simulink model "SITL_gerador_codigo"  (R2015a)
settings: Solver=FixedStepDiscrete  StartTime=0.0  StopTime=tempofinal  FixedStep=Td  RelTol=1e-3
values from neighbouring files (symbols this model uses):
  cq = 2.4086*10^(-7)    (= 2.4086e-07)    [main_quad.m]
  ct = 1.4341*10^(-5)    (= 1.4341e-05)    [main_quad.m]
  d = 0.26    [main_quad.m]
  g = 9.8065    [main_quad.m]
  J = [Jxx,Jyy,Jzz,Jm]    [main_quad.m]
  k1 = 2.5    [main_quad.m]
  k2 = 6.2360    (= 6.236)    [main_quad.m]
  k3 = 6.2360    (= 6.236)    [main_quad.m]
  k4 = 0.4927    [main_quad.m]
  k5 = 1.6    [main_quad.m]
  k6 = 1.6    [main_quad.m]
  lambda1 = 1    [main_quad.m]
  lambda2 = 5    [main_quad.m]
  lambda3 = 5    [main_quad.m]
  lambda4 = 1/2    (= 0.5)    [main_quad.m]
  lambda5 = 1/4    (= 0.25)    [main_quad.m]
  lambda6 = 1/4    (= 0.25)    [main_quad.m]
  limit = [0.5 0.5 0.5 0.5]    [main_quad.m]
  limit_pos = [0.5 0.5]    [main_quad.m]
  m = 1.03    [main_quad.m]
  X = A(:,1)    [plot_resultados.m]
undefined symbols (not defined in the file or in its folder): selecting_parameters
libraries: dspnetwork x2, etargetslib x2
settings Model: ParamWorkspaceSource=ReferencedWorkspace  ExtModeTrigDuration=100  TunableVars=J,Td,cq,ct,d,g,k1,k2,k3,k4,k5,k6,lambda1,lambda2,lambda3,lambda4,lambda5,lambda6,limit,limit_pos,m  TunableVarsStorageClass=Auto,Auto,Auto,Auto,Auto,Auto,Auto,Auto,Auto,Auto,Auto,Auto,Auto,Auto,Auto,Auto,Auto,Auto,Auto,Auto,Auto  TunableVarsTypeQualifier=,,,,,,,,,,,,,,,,,,,,  Creator=Adriano  LastModifiedBy=Andre
settings OptimizationCC: InlineParams=on  EnhancedBackFolding=on  CachingGlobalReferences=on  StrengthReduction=on  OptimizeModelRefInitCode=on  LifeSpan=1  SimCompilerOptimization=on
settings DebuggingCC: UnderspecifiedInitializationDetection=Classic  MergeDetectMultiDrivingBlocksExec=none  SolverPrmCheckMsg=warning  StateNameClashWarn=warning
settings HardwareCC: ProdLargestAtomicInteger=Long  ProdLargestAtomicFloat=Double  ProdIntDivRoundTo=Zero  ProdEndianess=LittleEndian  ProdHWDeviceType=ARM Compatible->ARM Cortex
settings RTWCC: SystemTargetFile=ert.tlc  GenCodeOnly=on  GenerateMakefile=off  TemplateMakefile=ert_default_tmf  Description=Embedded Coder  GenerateReport=on  RTWVerbose=off  IncludeHyperlinkInReport=on  LaunchReport=on  RTWCompilerOptimization=on  CheckMdlBeforeBuild=Warning
settings CodeAppCC: IgnoreCustomStorageClasses=off
settings ERTTargetCC: ParMdlRefBuildCompliant=on  CompOptLevelCompliant=on  ConcurrentExecutionCompliant=on  ERTFirstTimeCompliant=on  SupportContinuousTime=off  SupportVariableSizeSignals=off  ModelStepFunctionPrototypeControlCompliant=on  CPPClassGenCompliant=on  InlinedParameterPlacement=Hierarchical  ERTCustomFileTemplate=example_file_process.tlc

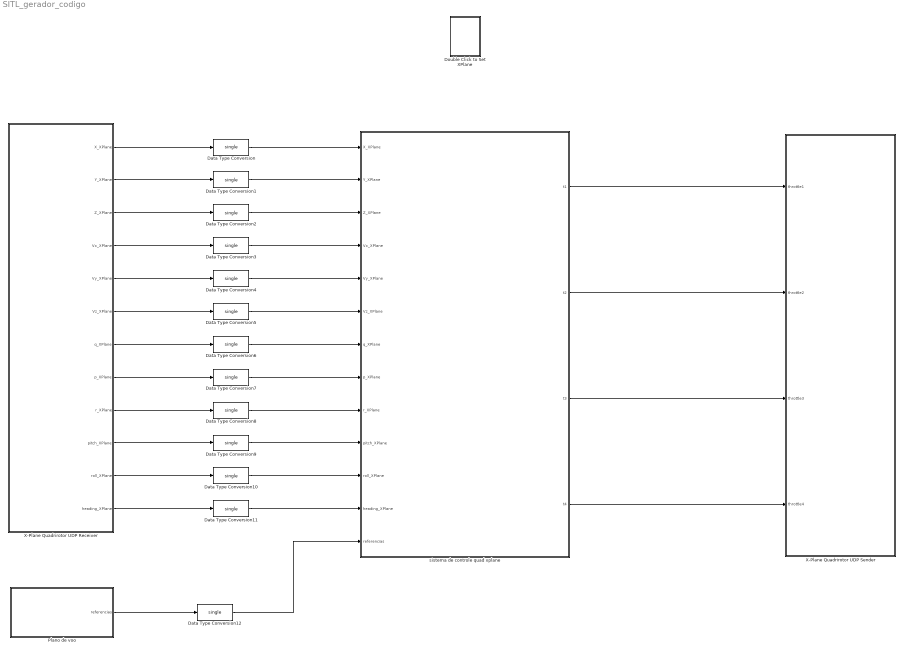
== system SITL_gerador_codigo ==
  Data Type Conversion{,1..12} (13 alike) : DataTypeConversion  OutDataTypeStr=single
  Double Click to Set XPlane : Subsystem  LoadFcn=selecting_parameters()
      settings: OpenFcn=selecting_parameters()
  Plano de voo : Subsystem
  X-Plane Quadrirotor UDP Receiver : Subsystem  AncestorBlock=X_Plane_Communication_Library/Fixed Wing/X-Plane Fixed Wing UDP Receiver  mask{ip_adress='127.0.0.1', port_number=49004}
      mask prompts: ip_adress "Local IP Adress (default: '127.0.0.1' )"; port_number "Output Port Number (defaut: '49004')"
      mask help: This block is configured to receiver data from a fixed wing aircraft on X-Plane Flight Simulator.
      mask Help: Contact adrianobittar@gmail.com
  X-Plane Quadrirotor UDP Sender : Subsystem  AncestorBlock=X_Plane_Communication_Library/Fixed Wing/X-Plane Fixed Wing UDP Sender  mask{ip_adress='127.0.0.1', port_number=49000}
      mask prompts: ip_adress "Local IP Adress (default: '127.0.0.1' )"; port_number "Output Port Number (defaut: '49000')"
      mask help: This block is configured to send data to a fixed wing aircraft on X-Plane Flight Simulator.
      mask Help: Contact adrianobittar@gmail.com
  sistema de controle quad xplane : Subsystem  DataTypeOverride=Single
  wires:
  X-Plane Quadrirotor UDP Receiver/1("X_XPlane ") -> Data Type Conversion/1
  X-Plane Quadrirotor UDP Receiver/2(Y_XPlane) -> Data Type Conversion1/1
  X-Plane Quadrirotor UDP Receiver/3(Z_XPlane) -> Data Type Conversion2/1
  X-Plane Quadrirotor UDP Receiver/4(Vx_XPlane) -> Data Type Conversion3/1
  X-Plane Quadrirotor UDP Receiver/5(Vy_XPlane) -> Data Type Conversion4/1
  X-Plane Quadrirotor UDP Receiver/6(Vz_XPlane) -> Data Type Conversion5/1
  X-Plane Quadrirotor UDP Receiver/7(q_XPlane) -> Data Type Conversion6/1
  X-Plane Quadrirotor UDP Receiver/8(p_XPlane) -> Data Type Conversion7/1
  X-Plane Quadrirotor UDP Receiver/9(r_XPlane) -> Data Type Conversion8/1
  X-Plane Quadrirotor UDP Receiver/10(pitch_XPlane) -> Data Type Conversion9/1
  X-Plane Quadrirotor UDP Receiver/11(roll_XPlane) -> Data Type Conversion10/1
  X-Plane Quadrirotor UDP Receiver/12(heading_XPlane) -> Data Type Conversion11/1
  Plano de voo/1("referencias ") -> Data Type Conversion12/1
  sistema de controle quad xplane/1(t1) -> X-Plane Quadrirotor UDP Sender/1(throttle1)
  sistema de controle quad xplane/2(t2) -> X-Plane Quadrirotor UDP Sender/2(throttle2)
  sistema de controle quad xplane/3(t3) -> X-Plane Quadrirotor UDP Sender/3(throttle3)
  sistema de controle quad xplane/4(t4) -> X-Plane Quadrirotor UDP Sender/4(throttle4)
  Data Type Conversion/1 -> sistema de controle quad xplane/1(X_XPlane)
  Data Type Conversion1/1 -> sistema de controle quad xplane/2(Y_XPlane)
  Data Type Conversion2/1 -> sistema de controle quad xplane/3(Z_XPlane)
  Data Type Conversion3/1 -> sistema de controle quad xplane/4(Vx_XPlane)
  Data Type Conversion4/1 -> sistema de controle quad xplane/5(Vy_XPlane)
  Data Type Conversion6/1 -> sistema de controle quad xplane/7(q_XPlane)
  Data Type Conversion5/1 -> sistema de controle quad xplane/6(Vz_XPlane)
  Data Type Conversion7/1 -> sistema de controle quad xplane/8(p_XPlane)
  Data Type Conversion9/1 -> sistema de controle quad xplane/10(pitch_XPlane)
  Data Type Conversion8/1 -> sistema de controle quad xplane/9(r_XPlane)
  Data Type Conversion10/1 -> sistema de controle quad xplane/11(roll_XPlane)
  Data Type Conversion11/1 -> sistema de controle quad xplane/12(heading_XPlane)
  Data Type Conversion12/1 -> sistema de controle quad xplane/13(referencias)

== system SITL_gerador_codigo/Double Click to Set XPlane ==

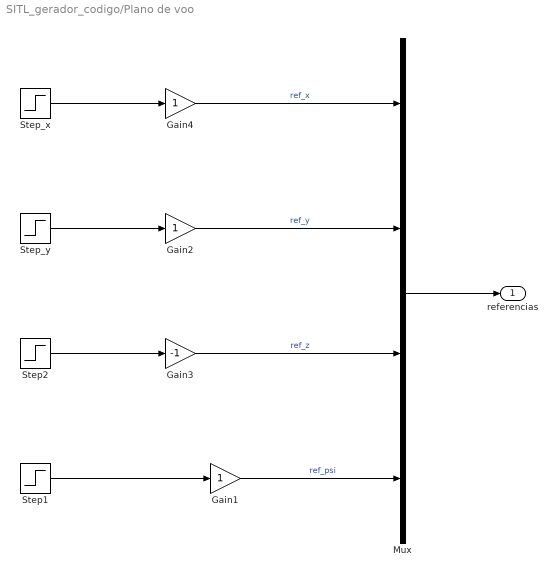
== system SITL_gerador_codigo/Plano de voo ==
  Gain1 : Gain
  Gain2 : Gain
  Gain3 : Gain  Gain=-1
  Gain4 : Gain
  Mux : Mux
  Step1 : Step  Time=30  After=150*pi/180  SampleTime=0
  Step2 : Step  Time=0  After=6  SampleTime=0
  Step_x : Step  Time=20  After=15  SampleTime=0
  Step_y : Step  Time=10  After=15  SampleTime=0
  "referencias " : Outport
  wires:
  Mux/1 -> "referencias "/1
  Gain3/1 -> Mux/3  "ref_z"
  Gain2/1 -> Mux/2  "ref_y"
  Gain4/1 -> Mux/1  "ref_x"
  Gain1/1 -> Mux/4  "ref_psi"
  Step1/1 -> Gain1/1
  Step2/1 -> Gain3/1
  Step_y/1 -> Gain2/1
  Step_x/1 -> Gain4/1

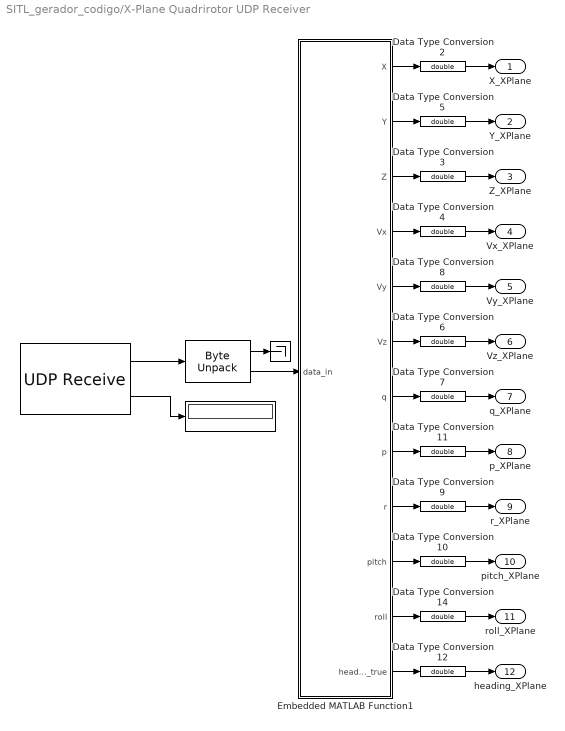
== system SITL_gerador_codigo/X-Plane Quadrirotor UDP Receiver ==
  " " : Display
  " " : Terminator
  "    " : dspnetwork/UDP Receive  localURL='0.0.0.0'  localPort=port_number  remoteURL=ip_adress  remotePort=-1  recvBufferSize=8192  dims=113  signalDatatype=uint8  isVarSize=off  showBlockingTime=on  blockingTime=1  sampletime=0.02  blockPlatform=WINDOWS
  "     " : etargetslib/Byte Unpack  dimensions={5,[9,3]}  datatypes={'uint8','single'}  byteAlign=1
  Data Type Conversion{2..12,14} (12 alike) : DataTypeConversion  OutDataTypeStr=double  SaturateOnIntegerOverflow=on
  Embedded MATLAB Function1 : MATLAB Function  TreatAsAtomicUnit=on
  "X_XPlane " : Outport
  Y_XPlane : Outport  Port=2
  Z_XPlane : Outport  Port=3
  Vx_XPlane : Outport  Port=4
  Vy_XPlane : Outport  Port=5
  Vz_XPlane : Outport  Port=6
  q_XPlane : Outport  Port=7
  p_XPlane : Outport  Port=8
  r_XPlane : Outport  Port=9
  pitch_XPlane : Outport  Port=10
  roll_XPlane : Outport  Port=11
  heading_XPlane : Outport  Port=12
  wires:
  Data Type Conversion11/1 -> p_XPlane/1
  Data Type Conversion14/1 -> roll_XPlane/1
  Data Type Conversion12/1 -> heading_XPlane/1
  Data Type Conversion7/1 -> q_XPlane/1
  Data Type Conversion6/1 -> Vz_XPlane/1
  Data Type Conversion4/1 -> Vx_XPlane/1
  Data Type Conversion3/1 -> Z_XPlane/1
  Data Type Conversion8/1 -> Vy_XPlane/1
  Data Type Conversion5/1 -> Y_XPlane/1
  Data Type Conversion2/1 -> "X_XPlane "/1
  Embedded MATLAB Function1/1(X) -> Data Type Conversion2/1
  Embedded MATLAB Function1/2(Y) -> Data Type Conversion5/1
  Embedded MATLAB Function1/3(Z) -> Data Type Conversion3/1
  Embedded MATLAB Function1/4(Vx) -> Data Type Conversion4/1
  Embedded MATLAB Function1/5(Vy) -> Data Type Conversion8/1
  Embedded MATLAB Function1/6(Vz) -> Data Type Conversion6/1
  Embedded MATLAB Function1/7(q) -> Data Type Conversion7/1
  Embedded MATLAB Function1/8(p) -> Data Type Conversion11/1
  Embedded MATLAB Function1/9(r) -> Data Type Conversion9/1
  Embedded MATLAB Function1/10(pitch) -> Data Type Conversion10/1
  Embedded MATLAB Function1/11(roll) -> Data Type Conversion14/1
  Embedded MATLAB Function1/12(heading_true) -> Data Type Conversion12/1
  "     "/1 -> " "/1
  "    "/2 -> " "/1
  Data Type Conversion10/1 -> pitch_XPlane/1
  "    "/1 -> "     "/1
  Data Type Conversion9/1 -> r_XPlane/1
  "     "/2 -> Embedded MATLAB Function1/1(data_in)

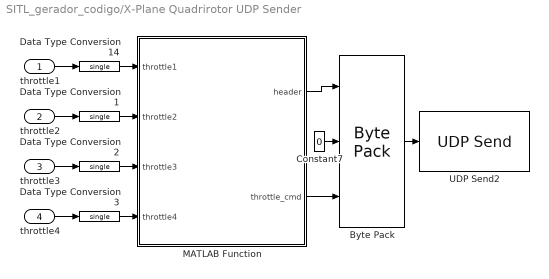
== system SITL_gerador_codigo/X-Plane Quadrirotor UDP Sender ==
  throttle1 : Inport
  throttle2 : Inport  Port=2
  throttle3 : Inport  Port=3
  throttle4 : Inport  Port=4
  Byte Pack : etargetslib/Byte Pack  datatypes={'single','uint8','single'}  byteAlign=1
  Constant7 : Constant  Value=0  OutDataTypeStr=uint8
  Data Type Conversion{1..3,14} (4 alike) : DataTypeConversion  OutDataTypeStr=single  SaturateOnIntegerOverflow=on
  MATLAB Function : MATLAB Function  TreatAsAtomicUnit=on
  UDP Send2 : dspnetwork/UDP Send  remoteURL=ip_adress  remotePort=port_number  localURL='255.255.255.255'  localPortSource=Automatically determine  localPort=-1  sampletime=-1  blockPlatform=HOST  separateLengthPort=0
  wires:
  Byte Pack/1 -> UDP Send2/1
  MATLAB Function/1(header) -> Byte Pack/1
  Data Type Conversion14/1 -> MATLAB Function/1(throttle1)
  throttle1/1 -> Data Type Conversion14/1
  Constant7/1 -> Byte Pack/2
  Data Type Conversion1/1 -> MATLAB Function/2(throttle2)
  Data Type Conversion2/1 -> MATLAB Function/3(throttle3)
  Data Type Conversion3/1 -> MATLAB Function/4(throttle4)
  throttle2/1 -> Data Type Conversion1/1
  throttle3/1 -> Data Type Conversion2/1
  throttle4/1 -> Data Type Conversion3/1
  MATLAB Function/2(throttle_cmd) -> Byte Pack/3

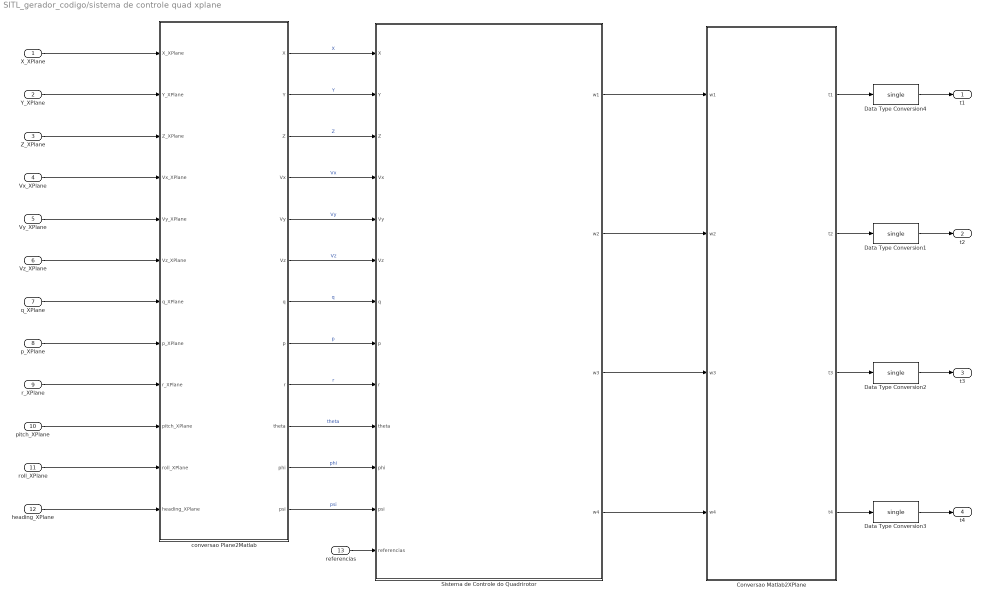
== system SITL_gerador_codigo/sistema de controle quad xplane ==
  X_XPlane : Inport
  Y_XPlane : Inport  Port=2
  Z_XPlane : Inport  Port=3
  Vx_XPlane : Inport  Port=4
  Vy_XPlane : Inport  Port=5
  Vz_XPlane : Inport  Port=6
  q_XPlane : Inport  Port=7
  p_XPlane : Inport  Port=8
  r_XPlane : Inport  Port=9
  pitch_XPlane : Inport  Port=10
  roll_XPlane : Inport  Port=11
  heading_XPlane : Inport  Port=12
  referencias : Inport  Port=13
  Conversao Matlab2XPlane : Subsystem
  Data Type Conversion{1..4} (4 alike) : DataTypeConversion  OutDataTypeStr=single
  Sistema de Controle do Quadrirotor : Subsystem
  conversao Plane2Matlab : Subsystem
  t1 : Outport
  t2 : Outport  Port=2
  t3 : Outport  Port=3
  t4 : Outport  Port=4
  wires:
  pitch_XPlane/1 -> conversao Plane2Matlab/10(pitch_XPlane)
  X_XPlane/1 -> conversao Plane2Matlab/1(X_XPlane)
  Y_XPlane/1 -> conversao Plane2Matlab/2(Y_XPlane)
  Z_XPlane/1 -> conversao Plane2Matlab/3(Z_XPlane)
  Vx_XPlane/1 -> conversao Plane2Matlab/4(Vx_XPlane)
  Vy_XPlane/1 -> conversao Plane2Matlab/5(Vy_XPlane)
  p_XPlane/1 -> conversao Plane2Matlab/8(p_XPlane)
  roll_XPlane/1 -> conversao Plane2Matlab/11(roll_XPlane)
  r_XPlane/1 -> conversao Plane2Matlab/9(r_XPlane)
  Vz_XPlane/1 -> conversao Plane2Matlab/6(Vz_XPlane)
  heading_XPlane/1 -> conversao Plane2Matlab/12(heading_XPlane)
  q_XPlane/1 -> conversao Plane2Matlab/7(q_XPlane)
  Sistema de Controle do Quadrirotor/3(w3) -> Conversao Matlab2XPlane/3(w3)
  Sistema de Controle do Quadrirotor/4(w4) -> Conversao Matlab2XPlane/4(w4)
  Sistema de Controle do Quadrirotor/2(w2) -> Conversao Matlab2XPlane/2(w2)
  Sistema de Controle do Quadrirotor/1(w1) -> Conversao Matlab2XPlane/1(w1)
  conversao Plane2Matlab/12(psi) -> Sistema de Controle do Quadrirotor/12(psi)  "psi"
  conversao Plane2Matlab/11(phi) -> Sistema de Controle do Quadrirotor/11(phi)  "phi"
  conversao Plane2Matlab/10(theta) -> Sistema de Controle do Quadrirotor/10(theta)  "theta"
  conversao Plane2Matlab/9(r) -> Sistema de Controle do Quadrirotor/9(r)  "r"
  conversao Plane2Matlab/8(p) -> Sistema de Controle do Quadrirotor/8(p)  "p"
  conversao Plane2Matlab/7(q) -> Sistema de Controle do Quadrirotor/7(q)  "q"
  conversao Plane2Matlab/6(Vz) -> Sistema de Controle do Quadrirotor/6(Vz)  "Vz"
  conversao Plane2Matlab/5(Vy) -> Sistema de Controle do Quadrirotor/5(Vy)  "Vy"
  conversao Plane2Matlab/4(Vx) -> Sistema de Controle do Quadrirotor/4(Vx)  "Vx"
  conversao Plane2Matlab/3(Z) -> Sistema de Controle do Quadrirotor/3(Z)  "Z"
  conversao Plane2Matlab/2(Y) -> Sistema de Controle do Quadrirotor/2(Y)  "Y"
  conversao Plane2Matlab/1("X ") -> Sistema de Controle do Quadrirotor/1(X)  "X"
  Conversao Matlab2XPlane/1(t1) -> Data Type Conversion4/1
  Conversao Matlab2XPlane/2(t2) -> Data Type Conversion1/1
  Conversao Matlab2XPlane/3(t3) -> Data Type Conversion2/1
  Conversao Matlab2XPlane/4(t4) -> Data Type Conversion3/1
  referencias/1 -> Sistema de Controle do Quadrirotor/13(referencias)
  Data Type Conversion4/1 -> t1/1
  Data Type Conversion1/1 -> t2/1
  Data Type Conversion2/1 -> t3/1
  Data Type Conversion3/1 -> t4/1

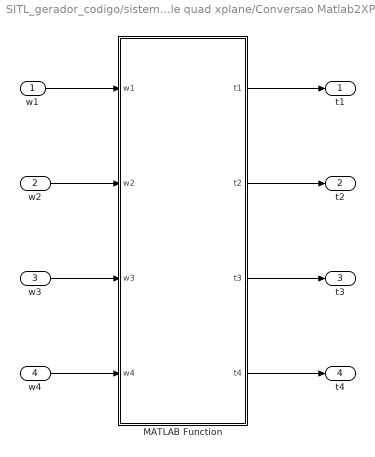
== system SITL_gerador_codigo/sistema de controle quad xplane/Conversao Matlab2XPlane ==
  w1 : Inport
  w2 : Inport  Port=2
  w3 : Inport  Port=3
  w4 : Inport  Port=4
  MATLAB Function : MATLAB Function  TreatAsAtomicUnit=on
  t1 : Outport
  t2 : Outport  Port=2
  t3 : Outport  Port=3
  t4 : Outport  Port=4
  wires:
  w1/1 -> MATLAB Function/1(w1)
  w2/1 -> MATLAB Function/2(w2)
  w3/1 -> MATLAB Function/3(w3)
  w4/1 -> MATLAB Function/4(w4)
  MATLAB Function/1(t1) -> t1/1
  MATLAB Function/2(t2) -> t2/1
  MATLAB Function/3(t3) -> t3/1
  MATLAB Function/4(t4) -> t4/1

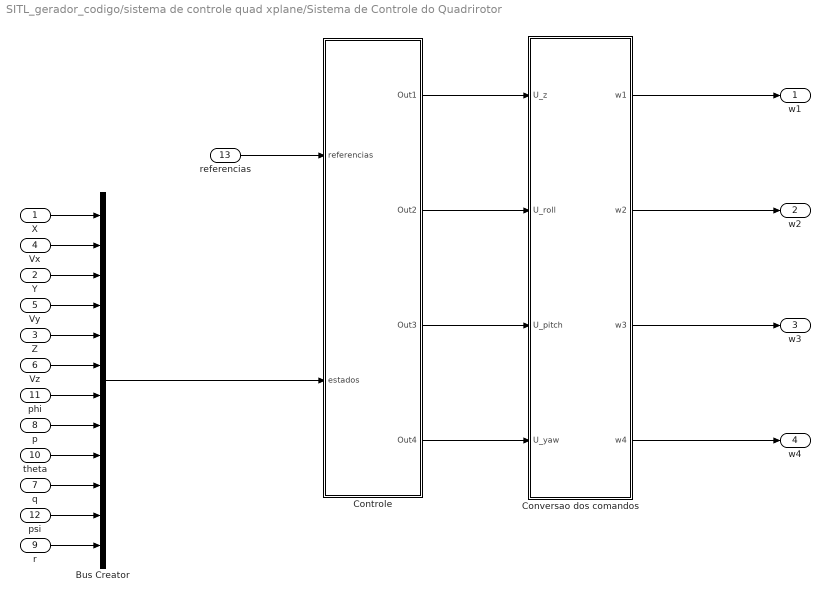
== system SITL_gerador_codigo/sistema de controle quad xplane/Sistema de Controle do Quadrirotor ==
  X : Inport
  Y : Inport  Port=2
  Z : Inport  Port=3
  Vx : Inport  Port=4
  Vy : Inport  Port=5
  Vz : Inport  Port=6
  q : Inport  Port=7
  p : Inport  Port=8
  r : Inport  Port=9
  theta : Inport  Port=10
  phi : Inport  Port=11
  psi : Inport  Port=12
  referencias : Inport  Port=13
  Bus Creator : BusCreator  Inputs=12
  Controle : Subsystem
  Conversao dos comandos : Subsystem
  w1 : Outport
  w2 : Outport  Port=2
  w3 : Outport  Port=3
  w4 : Outport  Port=4
  wires:
  Controle/1(Out1) -> Conversao dos comandos/1(U_z)
  Controle/2(Out2) -> Conversao dos comandos/2(U_roll)
  Controle/3(Out3) -> Conversao dos comandos/3(U_pitch)
  Controle/4(Out4) -> Conversao dos comandos/4(U_yaw)
  referencias/1 -> Controle/1(referencias)
  X/1 -> Bus Creator/1
  Bus Creator/1 -> Controle/2(estados)
  Vx/1 -> Bus Creator/2
  Y/1 -> Bus Creator/3
  Vy/1 -> Bus Creator/4
  Z/1 -> Bus Creator/5
  Vz/1 -> Bus Creator/6
  phi/1 -> Bus Creator/7
  p/1 -> Bus Creator/8
  theta/1 -> Bus Creator/9
  q/1 -> Bus Creator/10
  psi/1 -> Bus Creator/11
  r/1 -> Bus Creator/12
  Conversao dos comandos/1(w1) -> w1/1
  Conversao dos comandos/2(w2) -> w2/1
  Conversao dos comandos/3(w3) -> w3/1
  Conversao dos comandos/4(w4) -> w4/1

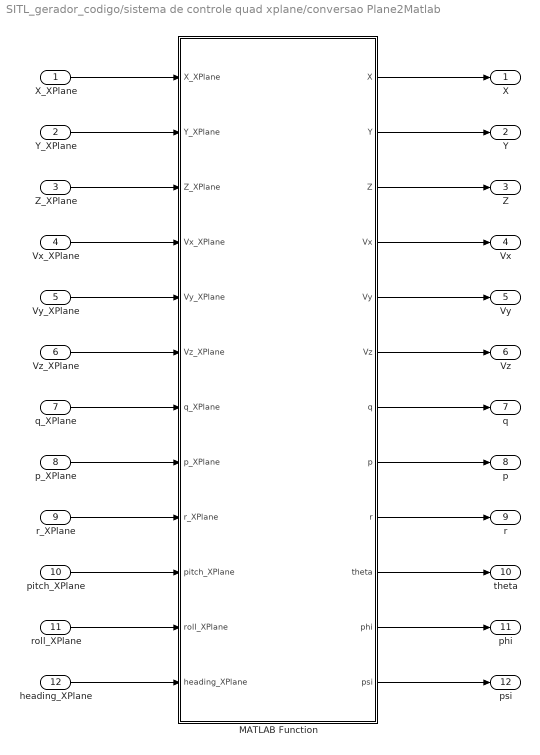
== system SITL_gerador_codigo/sistema de controle quad xplane/conversao Plane2Matlab ==
  X_XPlane : Inport
  Y_XPlane : Inport  Port=2
  Z_XPlane : Inport  Port=3
  Vx_XPlane : Inport  Port=4
  Vy_XPlane : Inport  Port=5
  Vz_XPlane : Inport  Port=6
  q_XPlane : Inport  Port=7
  p_XPlane : Inport  Port=8
  r_XPlane : Inport  Port=9
  pitch_XPlane : Inport  Port=10
  roll_XPlane : Inport  Port=11
  heading_XPlane : Inport  Port=12
  MATLAB Function : MATLAB Function  TreatAsAtomicUnit=on
  "X " : Outport
  Y : Outport  Port=2
  Z : Outport  Port=3
  Vx : Outport  Port=4
  Vy : Outport  Port=5
  Vz : Outport  Port=6
  q : Outport  Port=7
  p : Outport  Port=8
  r : Outport  Port=9
  theta : Outport  Port=10
  phi : Outport  Port=11
  psi : Outport  Port=12
  wires:
  MATLAB Function/12(psi) -> psi/1
  MATLAB Function/11(phi) -> phi/1
  MATLAB Function/10(theta) -> theta/1
  MATLAB Function/9(r) -> r/1
  MATLAB Function/8(p) -> p/1
  MATLAB Function/7(q) -> q/1
  MATLAB Function/6(Vz) -> Vz/1
  MATLAB Function/5(Vy) -> Vy/1
  MATLAB Function/4(Vx) -> Vx/1
  MATLAB Function/3(Z) -> Z/1
  MATLAB Function/2(Y) -> Y/1
  MATLAB Function/1(X) -> "X "/1
  X_XPlane/1 -> MATLAB Function/1(X_XPlane)
  Y_XPlane/1 -> MATLAB Function/2(Y_XPlane)
  Z_XPlane/1 -> MATLAB Function/3(Z_XPlane)
  Vx_XPlane/1 -> MATLAB Function/4(Vx_XPlane)
  Vy_XPlane/1 -> MATLAB Function/5(Vy_XPlane)
  Vz_XPlane/1 -> MATLAB Function/6(Vz_XPlane)
  q_XPlane/1 -> MATLAB Function/7(q_XPlane)
  p_XPlane/1 -> MATLAB Function/8(p_XPlane)
  r_XPlane/1 -> MATLAB Function/9(r_XPlane)
  pitch_XPlane/1 -> MATLAB Function/10(pitch_XPlane)
  roll_XPlane/1 -> MATLAB Function/11(roll_XPlane)
  heading_XPlane/1 -> MATLAB Function/12(heading_XPlane)

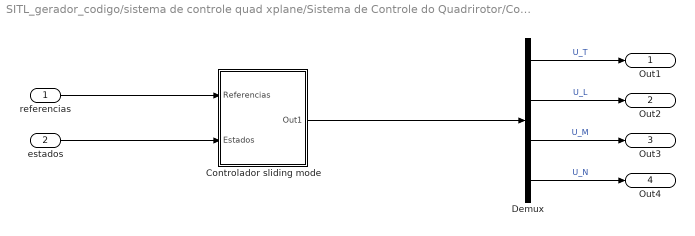
== system SITL_gerador_codigo/sistema de controle quad xplane/Sistema de Controle do Quadrirotor/Controle ==
  referencias : Inport
  estados : Inport  Port=2
  Controlador sliding mode : Subsystem
  Demux : Demux
  Out1 : Outport
  Out2 : Outport  Port=2
  Out3 : Outport  Port=3
  Out4 : Outport  Port=4
  wires:
  referencias/1 -> Controlador sliding mode/1(Referencias)
  estados/1 -> Controlador sliding mode/2(Estados)
  Controlador sliding mode/1(Out1) -> Demux/1
  Demux/1 -> Out1/1  "U_T"
  Demux/2 -> Out2/1  "U_L"
  Demux/3 -> Out3/1  "U_M"
  Demux/4 -> Out4/1  "U_N"

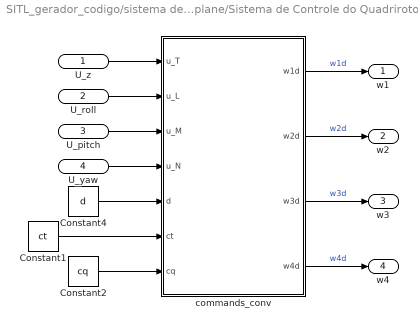
== system SITL_gerador_codigo/sistema de controle quad xplane/Sistema de Controle do Quadrirotor/Conversao dos comandos ==
  U_z : Inport
  U_roll : Inport  Port=2
  U_pitch : Inport  Port=3
  U_yaw : Inport  Port=4
  Constant1 : Constant  Value=ct  OutDataTypeStr=single
  Constant2 : Constant  Value=cq  OutDataTypeStr=single
  Constant4 : Constant  Value=d  OutDataTypeStr=single
  commands_conv : MATLAB Function  TreatAsAtomicUnit=on
  w1 : Outport
  w2 : Outport  Port=2
  w3 : Outport  Port=3
  w4 : Outport  Port=4
  wires:
  U_pitch/1 -> commands_conv/3(u_M)
  U_z/1 -> commands_conv/1(u_T)
  U_yaw/1 -> commands_conv/4(u_N)
  Constant4/1 -> commands_conv/5(d)
  Constant1/1 -> commands_conv/6(ct)
  Constant2/1 -> commands_conv/7(cq)
  U_roll/1 -> commands_conv/2(u_L)
  commands_conv/1(w1d) -> w1/1  "w1d"
  commands_conv/2(w2d) -> w2/1  "w2d"
  commands_conv/3(w3d) -> w3/1  "w3d"
  commands_conv/4(w4d) -> w4/1  "w4d"

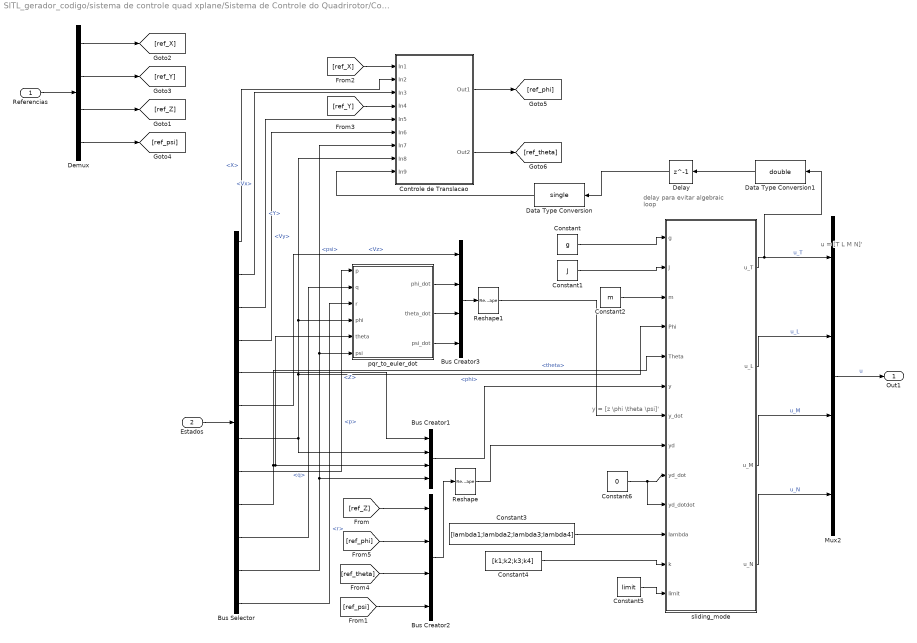
== system SITL_gerador_codigo/sistema de controle quad xplane/Sistema de Controle do Quadrirotor/Controle/Controlador sliding mode ==
  note: delay para evitar
      |  algebraic loop
  note: y = [z \phi \theta \psi]'
  note: u = [T L M N]'
  Referencias : Inport
  Estados : Inport  Port=2
  Bus Creator1 : BusCreator
  Bus Creator2 : BusCreator
  Bus Creator3 : BusCreator
  Bus Selector : BusSelector  OutputSignals=X,Vx,Y,Vy,Z,Vz,phi,p,theta,q,psi,r
  Constant : Constant  Value=g  OutDataTypeStr=single
  Constant1 : Constant  Value=J  OutDataTypeStr=single
  Constant2 : Constant  Value=m  OutDataTypeStr=single
  Constant3 : Constant  Value=[lambda1;lambda2;lambda3;lambda4]  OutDataTypeStr=single
  Constant4 : Constant  Value=[k1;k2;k3;k4]  OutDataTypeStr=single
  Constant5 : Constant  Value=limit  OutDataTypeStr=single
  Constant6 : Constant  Value=0  OutDataTypeStr=single
  Controle de Translacao : Subsystem
  Data Type Conversion : DataTypeConversion  OutDataTypeStr=single
  Data Type Conversion1 : DataTypeConversion  OutDataTypeStr=double
  Delay : Delay  DelayLength=1
  Demux : Demux
  Mux2 : Mux
  Reshape : Reshape  OutputDimensionality=Customize  OutputDimensions=[4,1]
  Reshape1 : Reshape  OutputDimensionality=Customize  OutputDimensions=[4,1]
  pqr_to_euler_dot : MATLAB Function  TreatAsAtomicUnit=on
  sliding_mode : MATLAB Function  TreatAsAtomicUnit=on
  Out1 : Outport
  wires:
  Demux/4 -> [ref_psi]
  Estados/1 -> Bus Selector/1
  Referencias/1 -> Demux/1
  Demux/1 -> [ref_X]
  Demux/2 -> [ref_Y]
  Demux/3 -> [ref_Z]
  Constant/1 -> sliding_mode/1(g)
  Constant1/1 -> sliding_mode/2(J)
  Constant2/1 -> sliding_mode/3(m)
  Bus Selector/5 -> Bus Creator1/1  "<Z>"
  Bus Selector/11 -> Bus Creator1/4, Controle de Translacao/7(In7), pqr_to_euler_dot/6(psi)  "<psi>"
  Constant3/1 -> sliding_mode/11(lambda)
  Constant4/1 -> sliding_mode/12(k)
  Mux2/1 -> Out1/1  "u"
  sliding_mode/1(u_T) -> Mux2/1, Data Type Conversion1/1  "u_T"
  sliding_mode/2(u_L) -> Mux2/2  "u_L"
  sliding_mode/4(u_N) -> Mux2/4  "u_N"
  sliding_mode/3(u_M) -> Mux2/3  "u_M"
  Bus Selector/2 -> Controle de Translacao/3(In3)  "<Vx>"
  Bus Selector/3 -> Controle de Translacao/5(In5)  "<Y>"
  Bus Selector/4 -> Controle de Translacao/6(In6)  "<Vy>"
  [ref_X] -> Controle de Translacao/1(In1)
  [ref_Y] -> Controle de Translacao/4(In4)
  [ref_Z] -> Bus Creator2/1
  [ref_psi] -> Bus Creator2/4
  Bus Creator2/1 -> Reshape/1
  [ref_theta] -> Bus Creator2/3
  [ref_phi] -> Bus Creator2/2
  Bus Creator1/1 -> sliding_mode/6(y)
  Controle de Translacao/1(Out1) -> [ref_phi]
  Controle de Translacao/2(Out2) -> [ref_theta]
  Reshape/1 -> sliding_mode/8(yd)
  Delay/1 -> Data Type Conversion/1
  Constant5/1 -> sliding_mode/13(limit)
  Bus Selector/6 -> Bus Creator3/1  "<Vz>"
  pqr_to_euler_dot/1(phi_dot) -> Bus Creator3/2
  pqr_to_euler_dot/2(theta_dot) -> Bus Creator3/3
  pqr_to_euler_dot/3(psi_dot) -> Bus Creator3/4
  Bus Creator3/1 -> Reshape1/1
  Reshape1/1 -> sliding_mode/7(y_dot)
  Bus Selector/1 -> Controle de Translacao/2(In2)  "<X>"
  Bus Selector/7 -> sliding_mode/4(Phi), pqr_to_euler_dot/4(phi), Controle de Translacao/8(In8), Bus Creator1/2  "<phi>"
  Bus Selector/12 -> pqr_to_euler_dot/3(r)  "<r>"
  Bus Selector/10 -> pqr_to_euler_dot/2(q)  "<q>"
  Bus Selector/8 -> pqr_to_euler_dot/1(p)  "<p>"
  Bus Selector/9 -> sliding_mode/5(Theta), pqr_to_euler_dot/5(theta), Bus Creator1/3  "<theta>"
  Data Type Conversion/1 -> Controle de Translacao/9(In9)
  Data Type Conversion1/1 -> Delay/1
  Constant6/1 -> sliding_mode/10(yd_dotdot), sliding_mode/9(yd_dot)

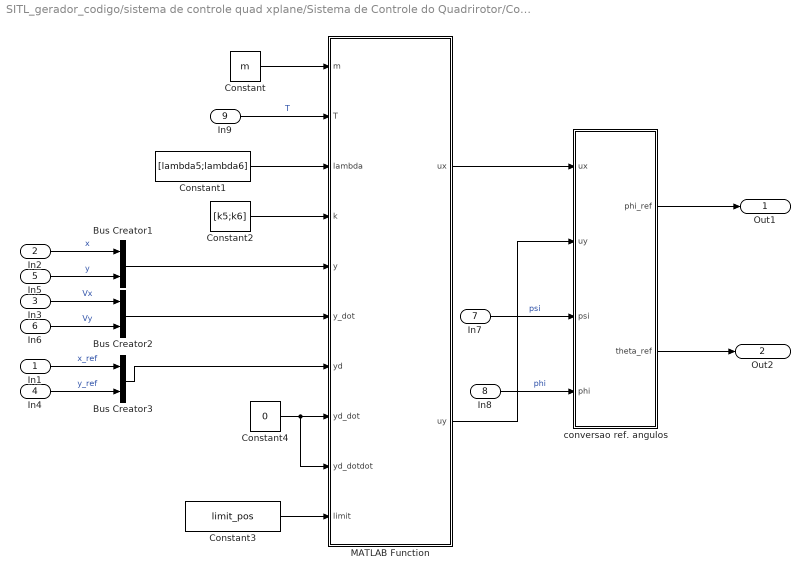
== system SITL_gerador_codigo/sistema de controle quad xplane/Sistema de Controle do Quadrirotor/Controle/Controlador sliding mode/Controle de Translacao ==
  In1 : Inport
  In2 : Inport  Port=2
  In3 : Inport  Port=3
  In4 : Inport  Port=4
  In5 : Inport  Port=5
  In6 : Inport  Port=6
  In7 : Inport  Port=7
  In8 : Inport  Port=8
  In9 : Inport  Port=9
  Bus Creator1 : BusCreator  Inputs=2
  Bus Creator2 : BusCreator  Inputs=2
  Bus Creator3 : BusCreator  Inputs=2
  Constant : Constant  Value=m  OutDataTypeStr=single
  Constant1 : Constant  Value=[lambda5;lambda6]  OutDataTypeStr=single
  Constant2 : Constant  Value=[k5;k6]  OutDataTypeStr=single
  Constant3 : Constant  Value=limit_pos  OutDataTypeStr=single
  Constant4 : Constant  Value=0  OutDataTypeStr=single
  MATLAB Function : MATLAB Function  TreatAsAtomicUnit=on
  conversao ref. angulos : MATLAB Function  TreatAsAtomicUnit=on
  Out1 : Outport
  Out2 : Outport  Port=2
  wires:
  conversao ref. angulos/1(phi_ref) -> Out1/1
  conversao ref. angulos/2(theta_ref) -> Out2/1
  Constant/1 -> MATLAB Function/1(m)
  Constant1/1 -> MATLAB Function/3(lambda)
  Constant2/1 -> MATLAB Function/4(k)
  Bus Creator1/1 -> MATLAB Function/5(y)
  In2/1 -> Bus Creator1/1  "x"
  In5/1 -> Bus Creator1/2  "y"
  Bus Creator2/1 -> MATLAB Function/6(y_dot)
  In3/1 -> Bus Creator2/1  "Vx"
  In6/1 -> Bus Creator2/2  "Vy"
  Bus Creator3/1 -> MATLAB Function/7(yd)
  In1/1 -> Bus Creator3/1  "x_ref"
  In4/1 -> Bus Creator3/2  "y_ref"
  In7/1 -> conversao ref. angulos/3(psi)  "psi"
  In8/1 -> conversao ref. angulos/4(phi)  "phi"
  In9/1 -> MATLAB Function/2(T)  "T"
  Constant3/1 -> MATLAB Function/10(limit)
  Constant4/1 -> MATLAB Function/9(yd_dotdot), MATLAB Function/8(yd_dot)
  MATLAB Function/1(ux) -> conversao ref. angulos/1(ux)
  MATLAB Function/2(uy) -> conversao ref. angulos/2(uy)

== matlab function SITL_gerador_codigo/X-Plane Quadrirotor UDP Receiver/Embedded MATLAB Function1 ==
  data: data_in input; X output; Y output; Z output; Vx output; Vy output; Vz output; q output; p output; r output; pitch output; roll output; heading_true output
function [X, Y, Z, Vx, Vy, Vz, q, p, r, pitch, roll, heading_true]   = fcn(data_in)

% data_in(a,b)
% a = number of the byte of the packet (the packet sent from X-Plane goes from 2 to 9, that are the intances)
% b = number of the the label selected on X-Plane (in this case it was selected 3 labels, so it goes from 1 to 3)

q = data_in(2,1);
p = data_in(3,1);
r = data_in(4,1);

pitch = data_in(2,2);
roll = data_in(3,2);
heading_true = data_in(4,2);

X = data_in(2,3);
Y = data_in(3,3);
Z = data_in(4,3);

Vx = data_in(5,3);
Vy = data_in(6,3);
Vz = data_in(7,3);

== matlab function SITL_gerador_codigo/sistema de controle quad xplane/Sistema de Controle do Quadrirotor/Conversao dos comandos/commands_conv ==
  data: u_T input single; w1d output single; u_L input single; u_M input single; u_N input single; w2d output single; w3d output single; w4d output single; d input single; ct input single; cq input single
function [w1d,w2d,w3d,w4d] = commands_conv(u_T,u_L,u_M,u_N,d,ct,cq)


u_z = u_T/(4*ct);
u_phi = u_L/(2*d*ct);
u_theta = u_M/(2*d*ct);
u_psi = u_N/(4*cq);

w1d_sq=u_z+u_theta+u_psi;
w2d_sq=u_z-u_phi-u_psi;
w3d_sq=u_z-u_theta+u_psi;
w4d_sq=u_z+u_phi-u_psi;


if w1d_sq<0
    w1d_sq=single(0);
end
if w2d_sq<0
    w2d_sq=single(0);
end
if w3d_sq<0
    w3d_sq=single(0);
end
if w4d_sq<0
    w4d_sq=single(0);
end

w1d = sqrt(w1d_sq);
w2d = sqrt(w2d_sq);
w3d = sqrt(w3d_sq);
w4d = sqrt(w4d_sq);

== matlab function SITL_gerador_codigo/X-Plane Quadrirotor UDP Sender/MATLAB Function ==
  data: throttle1 input; header output single size=1; throttle_cmd output size=[1 18]; throttle2 input; throttle3 input; throttle4 input
function [header, throttle_cmd]  = fcn(throttle1, throttle2, throttle3, throttle4)

%The header have 4 bytes plus one byte with 0

header = typecast(uint8([uint8(68) uint8(65) uint8(84) uint8(65)]), 'single');

%To send no comand for the instances we dont need to use, it is used -999

No_Comand = single(-999);

%The first group of four bytes in a selected field presents a label to identify the set of data(in this case throttle). 
%The second group has the first instance of the data set ;
%The third group has the second instance, etc. (Throttle1, 2, 3 and 4) 

Throttle_header = typecast(uint8([uint8(25) uint8(0) uint8(0) uint8(0)]), 'single');
throttle_cmd = [Throttle_header throttle1 throttle2 throttle3 throttle4 No_Comand No_Comand No_Comand No_Comand Throttle_header No_Comand No_Comand No_Comand No_Comand No_Comand No_Comand No_Comand No_Comand];

== matlab function SITL_gerador_codigo/sistema de controle quad xplane/Sistema de Controle do Quadrirotor/Controle/Controlador sliding mode/sliding_mode ==
  data: u_T output single; u_L output single; g input single; J input single; m input single; Phi input single; Theta input single; y input single; y_dot input single; yd input single; yd_dot input single; yd_dotdot input single; lambda input single; k input single; u_M output single; u_N output single; limit input single
function [u_T,u_L,u_M,u_N] = sliding_mode(g,J,m,Phi,Theta,y,y_dot,yd,yd_dot,yd_dotdot,lambda,k, limit)

Jxx=J(1);
Jyy=J(2);
Jzz=J(3);

lambdas = [lambda(1),0,0,0
          0,lambda(2),0,0
          0,0,lambda(3),0
          0,0,0,lambda(4)];

Phid = y_dot(2);
Thetad = y_dot(3);
Psid = y_dot(4);
      
f=zeros(4,1);

f(1)= g;

f(2)= cos(Phi)*tan(Theta)*(((Phid - Psid*sin(Theta))*(Jxx - Jyy)*(Thetad*cos(Phi) + ...
Psid*cos(Theta)*sin(Phi)))/Jzz) + sin(Phi)*tan(Theta)*(((Phid - Psid*sin(Theta))*(Jxx - Jzz)*(Thetad*sin(Phi) - Psid*cos(Phi)*cos(Theta)))/Jyy) + ...
(Psid*Thetad)/cos(Theta) + Phid*Thetad*tan(Theta) - ((Jyy - Jzz)*(Thetad*cos(Phi) + Psid*cos(Theta)*sin(Phi))*(Thetad*sin(Phi) - Psid*cos(Phi)*cos(Theta)))/Jxx;

f(3)= cos(Phi)*(((Phid - Psid*sin(Theta))*(Jxx - Jzz)*(Thetad*sin(Phi) - Psid*cos(Phi)*cos(Theta)))/Jyy) +...
    - sin(Phi)*(((Phid - Psid*sin(Theta))*(Jxx - Jyy)*(Thetad*cos(Phi) + Psid*cos(Theta)*sin(Phi)))/Jzz) - Phid*Psid*cos(Theta);

f(4) = (Phid*Thetad)/cos(Theta) + (cos(Phi)*(Jxx*(Phid - Psid*sin(Theta))*(Thetad*cos(Phi) + Psid*cos(Theta)*sin(Phi)) - Jyy*(Phid - Psid*sin(Theta))*(Thetad*cos(Phi) + Psid*cos(Theta)*sin(Phi))))/(Jzz*cos(Theta)) + ...
(sin(Phi)*(Jxx*(Phid - Psid*sin(Theta))*(Thetad*sin(Phi) - Psid*cos(Phi)*cos(Theta)) - Jzz*(Phid - Psid*sin(Theta))*(Thetad*sin(Phi) - Psid*cos(Phi)*cos(Theta))))/(Jyy*cos(Theta)) + (Psid*Thetad*sin(Theta))/cos(Theta);

s = y_dot - yd_dot + lambdas*(y - yd);


Binv=[-m/(cos(Phi)*cos(Theta)),0,0,0
       0, Jxx, 0,  -Jxx*sin(Theta)
       0, 0, (Jyy*cos(Phi)), (Jyy*cos(Theta)*sin(Phi))
       0, 0, -(Jzz*sin(Phi)), (Jzz*cos(Phi)*cos(Theta))];

k_des =  [k(1),0,0,0
          0,k(2),0,0
          0,0,k(3),0
          0,0,0,k(4)];
 
u = Binv * (-f + yd_dotdot - lambdas*(y_dot - yd_dot) - k_des * sat(s,limit));


u_T = u(1);
u_L = u(2);
u_M = u(3);
u_N = u(4);

== matlab function SITL_gerador_codigo/sistema de controle quad xplane/Sistema de Controle do Quadrirotor/Controle/Controlador sliding mode/pqr_to_euler_dot ==
  data: p input single; phi_dot output single; q input single; r input single; phi input single; theta input single; psi input single; theta_dot output single; psi_dot output
function [phi_dot,theta_dot,psi_dot] = pqr_to_euler_dot(p,q,r,phi,theta,psi)

phi_dot = p + tan(theta)*sin(phi)*q + tan(theta)*cos(phi)*r;

theta_dot = cos(phi)*q - sin(phi)*r;

psi_dot = q*sin(phi)/cos(theta) + r*cos(phi)/cos(theta);

== matlab function SITL_gerador_codigo/sistema de controle quad xplane/Sistema de Controle do Quadrirotor/Controle/Controlador sliding mode/Controle de Translacao/conversao ref. angulos ==
  data: ux input single; uy input single; psi input single; phi input single; phi_ref output single; theta_ref output single
function [phi_ref,theta_ref] = conv_ang_ref(ux,uy,psi,phi)

arg_phi = ux*sin(psi)-uy*cos(psi);


if arg_phi>1
    arg_phi=single(1);
elseif arg_phi<-1
    arg_phi=single(-1);
end

arg_theta = (ux*cos(psi)+uy*sin(psi))/(cos(phi));

if arg_theta>1
    arg_theta=single(1);
elseif arg_theta<-1
    arg_theta=single(-1);
end


phi_ref = asin(arg_phi);

theta_ref = asin(arg_theta);

== matlab function SITL_gerador_codigo/sistema de controle quad xplane/Sistema de Controle do Quadrirotor/Controle/Controlador sliding mode/Controle de Translacao/MATLAB Function ==
  data: m input single; T input single; lambda input single; k input single; y input single; y_dot input single; yd input single; yd_dot input single; yd_dotdot input single; ux output single; uy output single; limit input single
function [ux,uy] = posicao_sliding(m,T,lambda, k, y, y_dot, yd, yd_dot, yd_dotdot, limit)

lambdas=[lambda(1), 0
            0, lambda(2)];
        
k_des = [ k(1), 0 
             0, k(2)];
         
Binv= [-m/T, 0
        0, -m/T];
    
s = y_dot - yd_dot + lambdas*(y - yd);

u = Binv*(yd_dotdot - lambdas*(y_dot-yd_dot) - k_des*sat(s,limit));

ux=u(1);
uy=u(2);

== matlab function SITL_gerador_codigo/sistema de controle quad xplane/Conversao Matlab2XPlane/MATLAB Function ==
  data: w1 input; t1 output; w2 input; w3 input; w4 input; t2 output; t3 output; t4 output
function [t1,t2,t3,t4] = commands_conv(w1,w2,w3,w4)

% this block is responsible for convert the angular velocity of each motor calculated on
% the control system and make it compatible with X-Plane.


w1_rpm=1.725*(60/(2*pi))*w1; % Convertion from rad/s to rpm and multiplied by a constant to make it compatible with hover velocity of X-Plane.

%t1= 0.00000000000075*w1_rpm*w1_rpm*w1_rpm;
t1= 0.0000000045*w1_rpm*w1_rpm;  % Convertion from angular velocity of the motors to thrust command. This value is sent to X-Plane.
%t1= 0.0000342*w1_rpm;


w2_rpm=1.725*(60/(2*pi))*w2;

%t2= 0.00000000000075*w2_rpm*w2_rpm*w2_rpm;
t2= 0.0000000045*w2_rpm*w2_rpm;
%t2= 0.0000342*w2_rpm;


w3_rpm=1.725*(60/(2*pi))*w3;

%t3= 0.00000000000075*w3_rpm*w3_rpm*w3_rpm;
t3= 0.0000000045*w3_rpm*w3_rpm;
%t3= 0.0000342*w3_rpm;


w4_rpm=1.725*(60/(2*pi))*w4;

%t4= 0.00000000000075*w4_rpm*w4_rpm*w4_rpm;
t4= 0.0000000045*w4_rpm*w4_rpm;
%t4= 0.0000342*w4_rpm;

== matlab function SITL_gerador_codigo/sistema de controle quad xplane/conversao Plane2Matlab/MATLAB Function ==
  data: X_XPlane input single; X output single; Y_XPlane input single; Z_XPlane input single; Vx_XPlane input single; Y output single; Z output single; Vx output single; Vy output single; Vz output single; q output single; p output single; r output single; theta output single; phi output single; psi output single; Vy_XPlane input single; Vz_XPlane input single; q_XPlane input single; p_XPlane input single; r_XPlane input single; pitch_XPlane input single; roll_XPlane input single; heading_XPlane input single
function [X,Y,Z,Vx,Vy,Vz,q,p,r,theta,phi,psi] = commands_conv(X_XPlane,Y_XPlane,Z_XPlane,Vx_XPlane,Vy_XPlane,Vz_XPlane,q_XPlane,p_XPlane,r_XPlane,pitch_XPlane,roll_XPlane,heading_XPlane)

%this block is responsible to make the variables of Xplane compatible with
%the variables of the control system.

X0=-35162.53;  %Initial position of the Quadcopter on X-Plane 
Y0=180.60;     %TODO: Get the values autonomously
Z0=2784.36;


X=-Z_XPlane-(-Z0); % CONVERTION FOR NED SYSTEM
Y=X_XPlane-(X0);
Z=-Y_XPlane-(-Y0);

Vx=-Vz_XPlane; % CONVERTION FOR NED SYSTEM 
Vy=Vx_XPlane;
Vz=-Vy_XPlane;

q=q_XPlane; % EQUAL
p=p_XPlane;
r=r_XPlane;

theta=pitch_XPlane*(pi/180); % CONVERTION FROM DEG TO RAD
phi=roll_XPlane*(pi/180);
psi=heading_XPlane*(pi/180);
